simulink library "tank_model"  (R2016a)
settings: Solver=ode45  StartTime=0.0  StopTime=10.0  RelTol=1e-3
settings Model: Creator=Ibrahim  LastModifiedBy=Ibrahim
settings DataIOCC: LimitDataPoints=on
settings DebuggingCC: AllowSymbolicDim=off

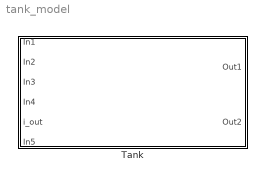
== system tank_model ==
  Tank : Subsystem

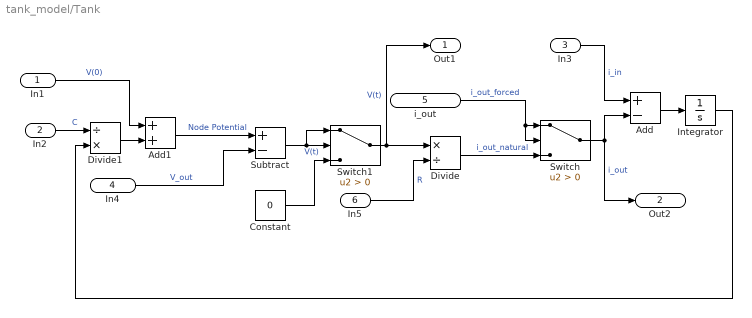
== system tank_model/Tank ==
  In1 : Inport
  In2 : Inport  Port=2
  In3 : Inport  Port=3
  In4 : Inport  Port=4
  i_out : Inport  Port=5
  In5 : Inport  Port=6
  Add : Sum  Inputs=+-
  Add1 : Sum
  Constant : Constant  Value=0
  Divide : Product  Inputs=*/
  Divide1 : Product  Inputs=/*
  Integrator : Integrator
  Subtract : Sum  Inputs=+-
  Switch : Switch  Criteria=u2 > Threshold
  Switch1 : Switch  Criteria=u2 > Threshold
  Out1 : Outport
  Out2 : Outport  Port=2
  wires:
  Add/1 -> Integrator/1
  In3/1 -> Add/1  "i_in"
  Integrator/1 -> Divide1/2
  In5/1 -> Divide/2  "R"
  Divide1/1 -> Add1/2
  Add1/1 -> Subtract/1  "Node Potential"
  In1/1 -> Add1/1  "V(0)"
  In2/1 -> Divide1/1  "C"
  Subtract/1 -> Switch1/1, Switch1/2  "V(t)"
  In4/1 -> Subtract/2  "V_out"
  Divide/1 -> Switch/3  "i_out_natural"
  i_out/1 -> Switch/2, Switch/1  "i_out_forced"
  Switch/1 -> Out2/1, Add/2  "i_out"
  Switch1/1 -> Divide/1, Out1/1  "V(t)"
  Constant/1 -> Switch1/3
